simulink model "LAB1__2_3"  (R2020a)
settings: Solver=VariableStepAuto  StartTime=0.0  StopTime=10.0  RelTol=1e-3
settings Model: Creator=Пользователь  LastModifiedBy=Пользователь

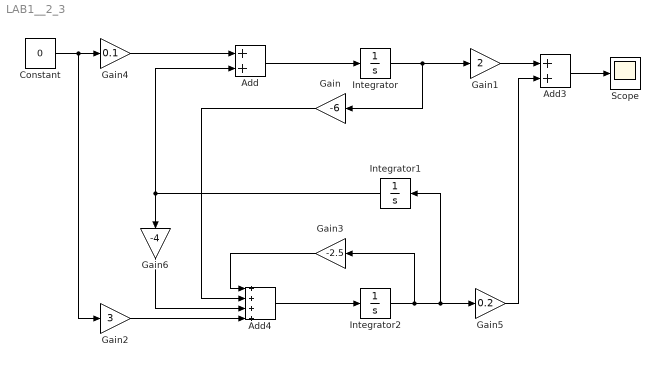
== system LAB1__2_3 ==
  Add : Sum
  Add3 : Sum
  Add4 : Sum  Inputs=++++
  Constant : Constant  Value=0
  Gain : Gain  Gain=-6
  Gain1 : Gain  Gain=2
  Gain2 : Gain  Gain=3
  Gain3 : Gain  Gain=-2.5
  Gain4 : Gain  Gain=0.1
  Gain5 : Gain  Gain=0.2
  Gain6 : Gain  Gain=-4
  Integrator : Integrator  InitialCondition=0.5
  Integrator1 : Integrator  InitialCondition=2
  Integrator2 : Integrator
  Scope : Scope
  wires:
  Gain3/1 -> Add4/1
  Gain/1 -> Add4/2
  Gain6/1 -> Add4/3
  Gain2/1 -> Add4/4
  Add3/1 -> Scope/1
  Gain5/1 -> Add3/2
  Integrator1/1 -> Gain6/1, Add/2
  Integrator2/1 -> Gain3/1, Gain5/1, Integrator1/1
  Add4/1 -> Integrator2/1
  Gain1/1 -> Add3/1
  Integrator/1 -> Gain1/1, Gain/1
  Add/1 -> Integrator/1
  Gain4/1 -> Add/1
  Constant/1 -> Gain4/1, Gain2/1
